simulink model "dc_buck_converter"  (R2021a)
settings: Solver=VariableStepAuto  StartTime=0.0  StopTime=0.2  FixedStep=1e-4  MaxStep=1e-4  RelTol=1e-4  EnableMultiTasking=on
undefined symbols (not defined in the file or in its folder): PARAMETERS
libraries: spsSeriesRLCBranchLib x5, spsMosfetLib x4, spsCurrentMeasurementLib x1, spsDiodeLib x1, spsPWMGeneratorDCDCLib x1, spsDCVoltageSourceLib x1, spsVoltageMeasurementLib x1, spspowerguiLib x1
settings Model: Creator=MathWorks  LastModifiedBy=jagprieto
settings SolverCC: AlgebraicLoopSolver=TrustRegion  SolverResetMethod=Robust
settings DataIOCC: ReturnWorkspaceOutputs=off
settings OptimizationCC: EfficientFloat2IntCast=on  LifeSpan=inf
settings DebuggingCC: UniqueDataStoreMsg=error  StrictBusMsg=ErrorOnBusTreatedAsVector  SFUnexpectedBacktrackingDiag=warning  SFNoUnconditionalDefaultTransitionDiag=warning  SFExecutionAtInitializationDiag=none  SFMachineParentedDataDiag=warning  ArithmeticOperatorsInVariantConditions=warning
settings SFSimCC: SimUseLocalCustomCode=off  CustomCodeUndefinedFunction=UseInterfaceOnly
settings RTWCC: RTWUseLocalCustomCode=off
settings CodeAppCC: StateflowObjectComments=on
settings GRTTargetCC: TargetLangStandard=C89/C90 (ANSI)
settings ConfigComp: CovMetricSettings=dw  CovSaveCumulativeToWorkspaceVar=on  CovSaveSingleToWorkspaceVar=on  CovExternalEMLEnable=off
settings SimscapeCC: SimscapeNormalizeSystem=off

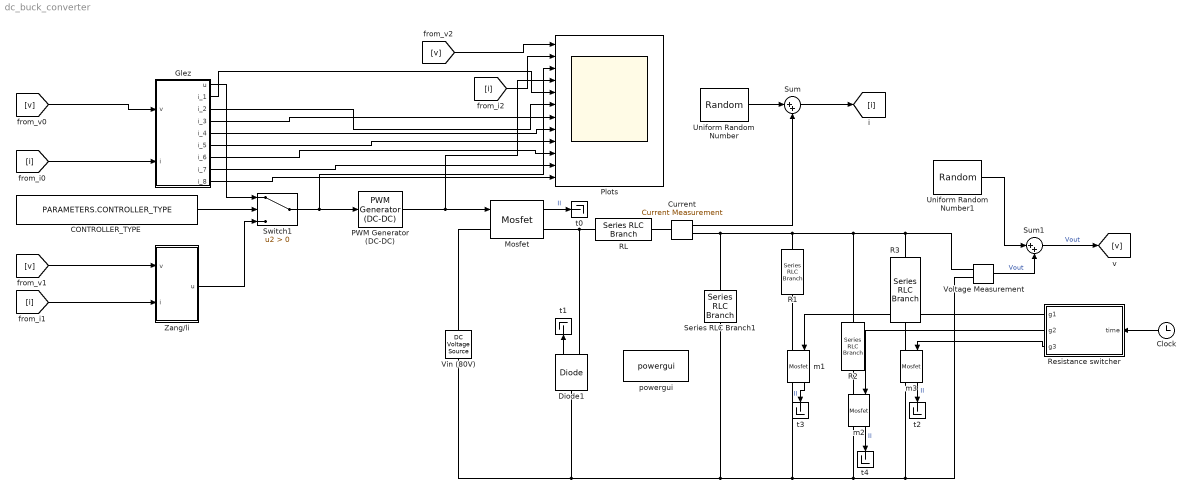
== system dc_buck_converter ==
  CONTROLLER_TYPE : Constant  Value=PARAMETERS.CONTROLLER_TYPE
  Clock : Clock
  Current : spsCurrentMeasurementLib/Current Measurement  PhasorSimulation=off  OutputType=Complex  PSBequivalent=0
  Diode1 : spsDiodeLib/Diode  Ron=1e-3  Lon=0  Vf=0  IC=0  UseSnubber=off  Rs=inf  Cs=inf  Measurements=on
  Glez : Subsystem  TreatAsAtomicUnit=on
  Mosfet : spsMosfetLib/Mosfet  Ron=1e-3  Lon=0  Rd=1e-3  Vfd=0  IC=0  Rs=inf  Cs=inf  Measurements=on
  PWM Generator (DC-DC) : spsPWMGeneratorDCDCLib/PWM Generator (DC-DC)  Fsw=PARAMETERS.SWITCHING_FREQUENCY  Ts=0
  Plots : Scope  NumInputPorts=12
  R1 : spsSeriesRLCBranchLib/Series RLC Branch  LConnTagsString=__new0  RConnTagsString=__new0  BranchType=R  Resistance=PARAMETERS.R  Inductance=1e-3  SetiL0=off  InitialCurrent=0  Capacitance=1e-6  Setx0=off  InitialVoltage=0  Measurements=None
  R2 : spsSeriesRLCBranchLib/Series RLC Branch  LConnTagsString=__new0  RConnTagsString=__new0  BranchType=R  Resistance=PARAMETERS.R2  Inductance=1e-3  SetiL0=off  InitialCurrent=0  Capacitance=1e-6  Setx0=off  InitialVoltage=0  Measurements=None
  R3 : spsSeriesRLCBranchLib/Series RLC Branch  LConnTagsString=__new0  RConnTagsString=__new0  BranchType=R  Resistance=PARAMETERS.R3  Inductance=1e-3  SetiL0=off  InitialCurrent=0  Capacitance=1e-6  Setx0=off  InitialVoltage=0  Measurements=None
  RL : spsSeriesRLCBranchLib/Series RLC Branch  LConnTagsString=__new0  RConnTagsString=__new0  BranchType=L  Resistance=0.02  Inductance=PARAMETERS.L  SetiL0=off  InitialCurrent=0  Capacitance=1e-6  Setx0=off  InitialVoltage=0  Measurements=None
  Resistance switcher : Subsystem
  Series RLC Branch1 : spsSeriesRLCBranchLib/Series RLC Branch  LConnTagsString=__new0  RConnTagsString=__new0  BranchType=C  Resistance=1e-4  Inductance=200e-6  SetiL0=off  InitialCurrent=0  Capacitance=PARAMETERS.C  Setx0=off  InitialVoltage=150  Measurements=None
  Sum : Sum  Inputs=|++
  Sum1 : Sum  Inputs=|++
  Switch1 : Switch  Criteria=u2 > Threshold
  Uniform Random Number : UniformRandomNumber  Minimum=-PARAMETERS.I_NOISE  Maximum=PARAMETERS.I_NOISE
  Uniform Random Number1 : UniformRandomNumber  Minimum=-PARAMETERS.V_NOISE  Maximum=PARAMETERS.V_NOISE
  Vin (80V) : spsDCVoltageSourceLib/DC Voltage Source  Amplitude=PARAMETERS.Vg  Measurements=None
  Voltage Measurement : spsVoltageMeasurementLib/Voltage Measurement  PhasorSimulation=off  OutputType=Complex  PSBequivalent=0
  Zang/li : Subsystem  TreatAsAtomicUnit=on
  m1 : spsMosfetLib/Mosfet  Ron=1e-6  Lon=0  Rd=1e-6  Vfd=0  IC=0  Rs=inf  Cs=inf  Measurements=on
  m2 : spsMosfetLib/Mosfet  Ron=1e-6  Lon=0  Rd=1e-6  Vfd=0  IC=0  Rs=inf  Cs=inf  Measurements=on
  m3 : spsMosfetLib/Mosfet  Ron=1e-6  Lon=0  Rd=1e-6  Vfd=0  IC=0  Rs=inf  Cs=inf  Measurements=on
  powergui : spspowerguiLib/powergui  Priority=1  SimulationMode=Continuous  SampleTime=PARAMETERS.SIMULATION_DT  frequency=60  Iterations=50  frequencyindice=0  Pbase=100e6  ErrMax=1e-4  UnitsV=kV  UnitsW=MW  buscounter=0  FunctionMessages=off  echomessages=off  EnableUseOfTLC=off  CurrentSourceSwitches=off  DisableSnubberDevices=off  DisableRonSwitches=off  DisableVfSwitches=off  DisplayEquations=off  AutomaticDiscreteSolvers=off  SolverType=Tustin/Backward Euler (TBE)  Interpol=off  ExternalGateDelay=off  methode=off  Ts=100  x0status=blocks  SPID=on  SwTol=0  HookPort=off  NonlinearTolerance=1e-4  nMaxIteration=100  ContinueOnMaxIteration=off  RestoreLinks=warning  ResistiveCurrentMeasurement=off  Frange=[0:2:500]  Ylog=off  Xlog=on  ShowGrid=off  save=off  variable=ZData  structure=0  ZoomFFT=off  StartTime=0.0  cycles=1  DisplayStyle=1  fundamental=60  FreqAxis=off  MaxFrequency=1000  frequencyindicesteady=1  RmsSteady=1  display=off
  t{0..4} (5 alike) : Terminator
  wires:
  Diode1/1 -> t1/1
  Mosfet/1 -> t0/1  "Il"
  Clock/1 -> Resistance switcher/1(time)
  CONTROLLER_TYPE/1 -> Switch1/2
  Zang/li/1(u) -> Switch1/3
  Resistance switcher/1(g1) -> m1/1
  Glez/1(u) -> Switch1/1
  m1/1 -> t3/1  "Il"
  m2/1 -> t4/1  "Il"
  Resistance switcher/2(g2) -> m2/1
  m3/1 -> t2/1  "Il"
  Resistance switcher/3(g3) -> m3/1
  Sum1/1 -> [v]  "Vout"
  Sum/1 -> [i]
  PWM Generator (DC-DC)/1 -> Plots/4, Mosfet/1
  Switch1/1 -> Plots/3, PWM Generator (DC-DC)/1
  [v] -> Glez/1(v)
  [v] -> Zang/li/1(v)
  [v] -> Plots/1
  [i] -> Glez/2(i)
  [i] -> Zang/li/2(i)
  [i] -> Plots/2
  Glez/2(i_1) -> Plots/5
  Glez/3(i_2) -> Plots/6
  Glez/4(i_3) -> Plots/7
  Glez/5(i_4) -> Plots/8
  Glez/6(i_5) -> Plots/9
  Glez/7(i_6) -> Plots/10
  Glez/8(i_7) -> Plots/11
  Glez/9(i_8) -> Plots/12
  Current/1 -> Sum/2
  Uniform Random Number/1 -> Sum/1
  Uniform Random Number1/1 -> Sum1/1
  Voltage Measurement/1 -> Sum1/2  "Vout"
  connections:
  Voltage Measurement/LConn2 -- m3/RConn1 -- m2/RConn1 -- Series RLC Branch1/RConn1 -- Diode1/LConn1 -- Vin (80V)/LConn1 -- m1/RConn1
  Series RLC Branch1/LConn1 -- Current/RConn1 -- R2/LConn1 -- R3/LConn1 -- Voltage Measurement/LConn1 -- R1/LConn1
  Vin (80V)/RConn1 -- Mosfet/LConn1
  Diode1/RConn1 -- RL/LConn1 -- Mosfet/RConn1
  Current/LConn1 -- RL/RConn1
  m1/LConn1 -- R1/RConn1
  m2/LConn1 -- R2/RConn1
  m3/LConn1 -- R3/RConn1

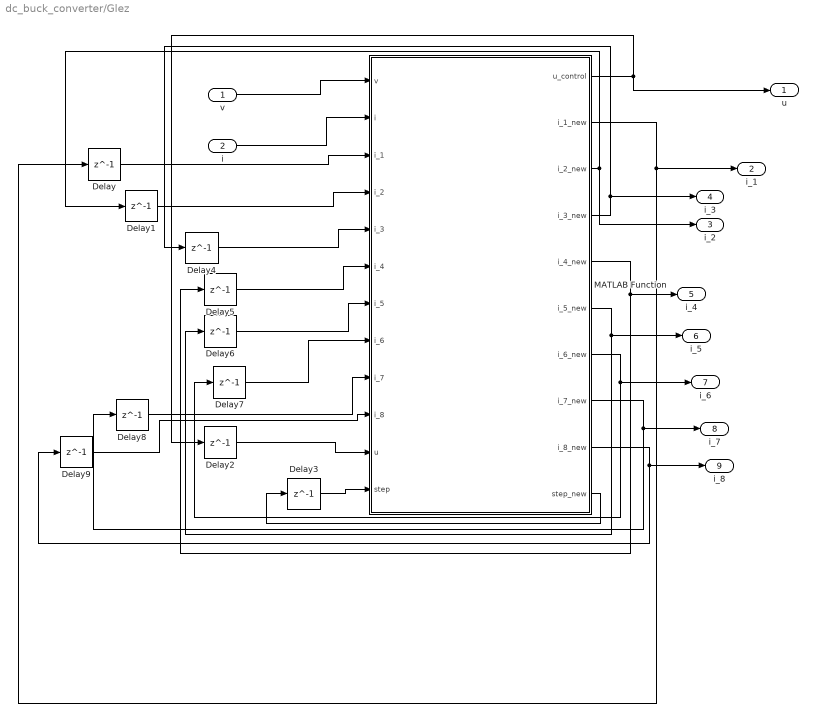
== system dc_buck_converter/Glez ==
  v : Inport
  i : Inport  Port=2
  Delay{,1..9} (10 alike) : Delay  DelayLength=1  InitialCondition=0
  MATLAB Function : MATLAB Function  TreatAsAtomicUnit=on  SystemSampleTime=PARAMETERS.SAMPLING_TIME
  u : Outport
  i_1 : Outport  Port=2
  i_2 : Outport  Port=3
  i_3 : Outport  Port=4
  i_4 : Outport  Port=5
  i_5 : Outport  Port=6
  i_6 : Outport  Port=7
  i_7 : Outport  Port=8
  i_8 : Outport  Port=9
  wires:
  v/1 -> MATLAB Function/1(v)
  i/1 -> MATLAB Function/2(i)
  Delay/1 -> MATLAB Function/3(i_1)
  MATLAB Function/2(i_1_new) -> Delay/1, i_1/1
  Delay1/1 -> MATLAB Function/4(i_2)
  MATLAB Function/3(i_2_new) -> i_2/1, Delay1/1
  Delay2/1 -> MATLAB Function/11(u)
  MATLAB Function/1(u_control) -> u/1, Delay2/1
  Delay4/1 -> MATLAB Function/5(i_3)
  MATLAB Function/4(i_3_new) -> i_3/1, Delay4/1
  Delay3/1 -> MATLAB Function/12(step)
  MATLAB Function/10(step_new) -> Delay3/1
  Delay5/1 -> MATLAB Function/6(i_4)
  MATLAB Function/5(i_4_new) -> i_4/1, Delay5/1
  Delay6/1 -> MATLAB Function/7(i_5)
  MATLAB Function/6(i_5_new) -> i_5/1, Delay6/1
  Delay7/1 -> MATLAB Function/8(i_6)
  MATLAB Function/7(i_6_new) -> i_6/1, Delay7/1
  Delay8/1 -> MATLAB Function/9(i_7)
  MATLAB Function/8(i_7_new) -> i_7/1, Delay8/1
  Delay9/1 -> MATLAB Function/10(i_8)
  MATLAB Function/9(i_8_new) -> i_8/1, Delay9/1

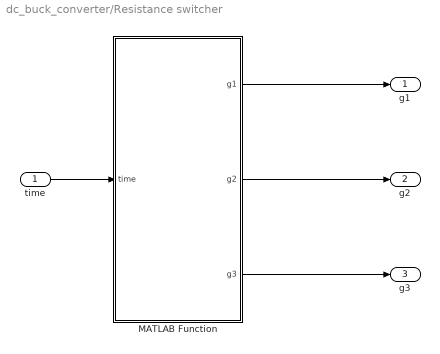
== system dc_buck_converter/Resistance switcher ==
  time : Inport
  MATLAB Function : MATLAB Function  TreatAsAtomicUnit=on  SystemSampleTime=PARAMETERS.SAMPLING_TIME
  g1 : Outport
  g2 : Outport  Port=2
  g3 : Outport  Port=3
  wires:
  MATLAB Function/1(g1) -> g1/1
  time/1 -> MATLAB Function/1(time)
  MATLAB Function/2(g2) -> g2/1
  MATLAB Function/3(g3) -> g3/1

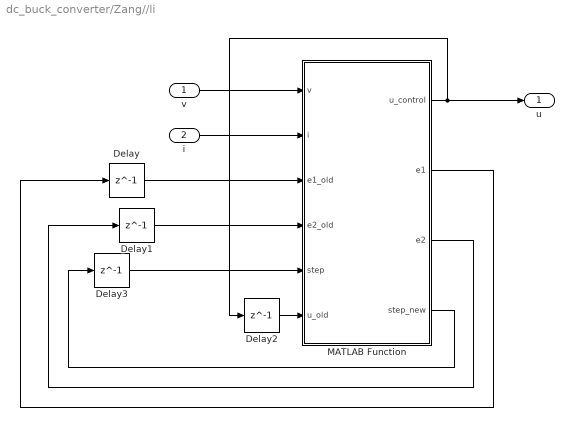
== system dc_buck_converter/Zang//li ==
  v : Inport
  i : Inport  Port=2
  Delay{,1..3} (4 alike) : Delay  DelayLength=1  InitialCondition=0
  MATLAB Function : MATLAB Function  TreatAsAtomicUnit=on  SystemSampleTime=PARAMETERS.SAMPLING_TIME
  u : Outport
  wires:
  v/1 -> MATLAB Function/1(v)
  i/1 -> MATLAB Function/2(i)
  Delay/1 -> MATLAB Function/3(e1_old)
  MATLAB Function/2(e1) -> Delay/1
  Delay1/1 -> MATLAB Function/4(e2_old)
  MATLAB Function/3(e2) -> Delay1/1
  Delay3/1 -> MATLAB Function/5(step)
  MATLAB Function/4(step_new) -> Delay3/1
  Delay2/1 -> MATLAB Function/6(u_old)
  MATLAB Function/1(u_control) -> Delay2/1, u/1

== matlab function dc_buck_converter/Resistance switcher/MATLAB Function ==
  data: g1 output; time input; PARAMETERS parameter; g2 output; g3 output
function [g1,g2,g3] = fcn(time, PARAMETERS)

if PARAMETERS.PROBLEM_TYPE == 0  % Con carga en arranque
    if time < 0.1
        g1 = 1;
        g2 = 0; 
        g3 = 0;
    elseif time < 0.3 
        g1 = 0;
        g2 = 1;
        g3 = 0;
    else
        g1 = 0;
        g2 = 0;
        g3 = 1;
    end
  
elseif PARAMETERS.PROBLEM_TYPE == 1 % Sin carga en arranque

    if time < 0.2
        g1 = 0;
        g2 = 0; 
        g3 = 0;
    elseif time < 0.3
        g1 = 1;
        g2 = 0;
        g3 = 0;
    elseif time < 0.4 
        g1 = 0;
        g2 = 1;
        g3 = 0;
    else
        g1 = 0;
        g2 = 0;
        g3 = 1;
    end
else
    g1 = 0;
    g2 = 0;
    g3 = 0;
end

== matlab function dc_buck_converter/Glez/MATLAB Function ==
  data: u_control output; v input; i input; i_1 input; i_2 input; i_3 input; i_4 input; i_5 input; i_6 input; i_7 input; i_8 input; u input; i_1_new output; PARAMETERS parameter; i_2_new output; i_3_new output; i_4_new output; i_5_new output; i_6_new output; i_7_new output; i_8_new output; step input; step_new output
function [u_control, i_1_new, i_2_new, i_3_new, i_4_new, i_5_new, i_6_new, i_7_new, i_8_new, step_new]= fcn(v, i, i_1, i_2, i_3, i_4, i_5, i_6, i_7, i_8, u, PARAMETERS, step)
   
    % Read parameters
    R = PARAMETERS.R;
    C = PARAMETERS.C;
    L = PARAMETERS.L;
    RC = R*C;

    % States (memory) read
    if (step == 0)
       v_est = v;
       i_est = i;
       epsilon_v = 0;
       epsilon_i = 0;
       exp_gain = -log(0.999/(PARAMETERS.CUT_OFF_FREQUENCY_MAX-PARAMETERS.CUT_OFF_FREQUENCY_MIN))/PARAMETERS.CURRENT_MAX;
       cut_off_frequency = (PARAMETERS.CUT_OFF_FREQUENCY_MAX-PARAMETERS.CUT_OFF_FREQUENCY_MIN)*exp(-exp_gain*abs(i)) + PARAMETERS.CUT_OFF_FREQUENCY_MIN;    
       dot_cut_off_frequency = 0.0;
    else
       v_est = i_1;
       i_est = i_2;
       epsilon_v = i_3;
       epsilon_i = i_4;
       cut_off_frequency = i_8;     
       dot_cut_off_frequency = i_6;
    end        
    gamma = 1 /(2*PARAMETERS.SAMPLING_TIME);
    
    % Voltage disturbance estimation
    lambda_zv = 2*PARAMETERS.CUT_OFF_FREQUENCY_DISTURBANCE_V;
    p2_zv = (5*lambda_zv^2+4)/(2*lambda_zv^3);
    beta_zv = lambda_zv / gamma;
    kappa_zv = beta_zv /(2*p2_zv);
    z_v = v - v_est;
    dot_epsilon_v = (lambda_zv^2/4)*z_v + kappa_zv*tanh(gamma*z_v);
    dist_v_est = lambda_zv*z_v + beta_zv*tanh(gamma*z_v) + epsilon_v;
    dot_v_est = (-v/(RC)) + i/C + dist_v_est;

    % Current disturbance estimation
    lambda_zi = 2*PARAMETERS.CUT_OFF_FREQUENCY_DISTURBANCE_I;
    p2_zi = (5*lambda_zi^2+4)/(2*lambda_zi^3);
    beta_zi = lambda_zi / gamma;
    kappa_zi = beta_zi /(2*p2_zi);
    z_i = i - i_est;
    dot_epsilon_i = (lambda_zi^2/4)*z_i + kappa_zi*tanh(gamma*z_i);
    dist_i_est = lambda_zi*z_i + beta_zi*tanh(gamma*z_i) + epsilon_i;

    % Current as virtual control    
    lambda_ev = 2*cut_off_frequency;
    dot_lambda_ev = 2*dot_cut_off_frequency;
    beta_ev = lambda_ev / gamma;  
    e_v = v - PARAMETERS.Vd;
    dot_e_v_est = dot_v_est - PARAMETERS.dd_Vd;
    i_c = C * ((v/RC) - dist_v_est + PARAMETERS.d_Vd - lambda_ev*e_v - beta_ev*tanh(gamma*e_v)); 
    dot_i_c_est = C * ((dot_v_est / RC) - dot_epsilon_v +  PARAMETERS.dd_Vd - lambda_ev*dot_e_v_est - beta_ev*((sech(gamma*e_v))^2)*dot_e_v_est - dot_lambda_ev*(e_v + ((tanh(gamma*e_v)/gamma))));

    % Voltage as current tracking control                
    e_i = i - i_c; 
    lambda_ei = 2*lambda_ev;
    beta_ei = lambda_ei / gamma;
    u_control = (L/PARAMETERS.Vg)*((v/L) - dist_i_est + dot_i_c_est - lambda_ei*e_i - beta_ei*tanh(gamma*e_i));  
    u_control = min(max(u_control, 0.0), 1.0);
    dot_i_est = -(v/L) + u_control*PARAMETERS.Vg/L + dist_i_est;        

    % Update cut-off frequency
    exp_gain = -log(0.999/(PARAMETERS.CUT_OFF_FREQUENCY_MAX-PARAMETERS.CUT_OFF_FREQUENCY_MIN))/PARAMETERS.CURRENT_MAX;
    cut_off_frequency = (PARAMETERS.CUT_OFF_FREQUENCY_MAX-PARAMETERS.CUT_OFF_FREQUENCY_MIN)*exp(-exp_gain*abs(i_est)) + PARAMETERS.CUT_OFF_FREQUENCY_MIN;        
    dot_cut_off_frequency = -exp_gain*(PARAMETERS.CUT_OFF_FREQUENCY_MAX-PARAMETERS.CUT_OFF_FREQUENCY_MIN)*exp(-exp_gain*abs(i_est))*sign(i_est)*dot_i_est;
    
    % Update states
    i_1_new = v_est + dot_v_est*PARAMETERS.SAMPLING_TIME;        
    i_2_new = i_est + dot_i_est*PARAMETERS.SAMPLING_TIME; 
    i_3_new = epsilon_v + dot_epsilon_v*PARAMETERS.SAMPLING_TIME; 
    i_4_new = epsilon_i + dot_epsilon_i*PARAMETERS.SAMPLING_TIME;  
    i_5_new = 0;   
    i_6_new = dot_cut_off_frequency;
    i_7_new = 0;  
    i_8_new = cut_off_frequency;
    step_new = step + 1;
    
end

== matlab function dc_buck_converter/Zang//li/MATLAB Function ==
  data: u_control output; v input; i input; e1_old input; e2_old input; step input; u_old input; e1 output; PARAMETERS parameter; e2 output; step_new output
function [u_control, e1, e2, step_new]= fcn(v, i, e1_old, e2_old, step, u_old, PARAMETERS)
k = 6.0e-3 / PARAMETERS.SETTLING_TIME;
c1 = 500*k;
c2 = 700*k;
alfa = 11/23;

LC = PARAMETERS.C*PARAMETERS.L;
RC =  PARAMETERS.C*PARAMETERS.R;
e1 = v - PARAMETERS.Vd;
e2 = (i/PARAMETERS.C) - (v/RC) - PARAMETERS.d_Vd;
d1 = ((e1 - e1_old)/PARAMETERS.SAMPLING_TIME) - e2_old;
d2 = - ((e2 - e2_old)/PARAMETERS.SAMPLING_TIME) - (e1_old/LC) ...
    - ((e2_old - PARAMETERS.d_Vd)/RC) - PARAMETERS.dd_Vd ...
    - 0.0*(PARAMETERS.Vg*u_old/LC) - 0.0*(PARAMETERS.Vd/LC); 

f_vd = -PARAMETERS.SAMPLING_TIME*PARAMETERS.Vd/LC + PARAMETERS.SAMPLING_TIME*PARAMETERS.d_Vd/RC - PARAMETERS.SAMPLING_TIME*PARAMETERS.dd_Vd;
e_sign = e1 + PARAMETERS.SAMPLING_TIME*e2 + PARAMETERS.SAMPLING_TIME*d1;
u_control = -(LC/(PARAMETERS.SAMPLING_TIME*PARAMETERS.Vg));
u_control = u_control*((c1-(PARAMETERS.SAMPLING_TIME/LC))*e1 + (PARAMETERS.SAMPLING_TIME*c1 + 1)*d1 ... 
            + c2*sign(e_sign)*((abs(e_sign))^alfa) + f_vd ...
            + (1.0 - (PARAMETERS.SAMPLING_TIME/RC) + (PARAMETERS.SAMPLING_TIME*c1))*e2 ...
            + PARAMETERS.SAMPLING_TIME*d2);
        
u_control = sign(u_control)*min(1.0, abs(u_control));
u_control = max(0.0, u_control);
step_new = step + 1;
